simulink model "AC_grid_Dynamic"  (R2025a)
settings: Solver=VariableStepAuto  StartTime=0.0  StopTime=10.0  RelTol=1e-3
undefined symbols (not defined in the file): C_Lines, Cbuses, fref, From_buses, From_nodes, L_Loads, Lines_fromM, Lines_toM, Load_buses, Nbuses, R_Lines, R_Loads, shift_lines, tap_lines, To_buses, To_nodes
(part 1 of 2)
settings Model: Creator=atomas  LastModifiedBy=atomas

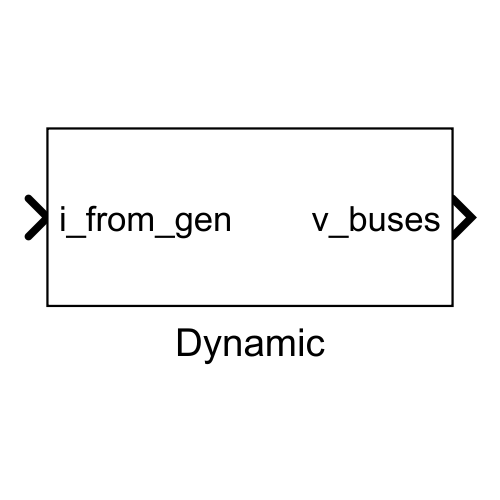
[thumbnail: Simulink's stored preview of the top-level diagram]
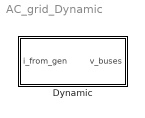
== system AC_grid_Dynamic ==
  Dynamic : Subsystem  VariantControl=Dynamic

== system AC_grid_Dynamic/Dynamic ==
  i_from_gen : Inport
  Buses : Subsystem
  Goto Tag Visibility : GotoTagVisibility  GotoTag=Cbuses
  Lines : Subsystem
  Lines to buses : Subsystem
  Loads : Subsystem
  Loads to buses : Subsystem
  Selector2 : Selector  NumberOfDimensions=2  InputPortWidth=Nnodes  IndexOptions=Select all,Index vector (dialog)  Indices=1,Load_buses  OutputSizes=1,1
  Selector4 : Selector  NumberOfDimensions=2  InputPortWidth=Nnodes  IndexOptions=Select all,Index vector (dialog)  Indices=From_nodes,From_buses  OutputSizes=1,1
  Selector6 : Selector  NumberOfDimensions=2  InputPortWidth=Nnodes  IndexOptions=Select all,Index vector (dialog)  Indices=To_nodes,To_buses  OutputSizes=1,1
  Step : Step  Before=ones(1, length(From_buses))  After=[1 ones(1, length(From_buses)-1)]  SampleTime=0
  Sum : Sum  Inputs=++|
  Sum1 : Sum  Inputs=|++
  connect : Subsystem
  iCbuses : Subsystem
  iP : Subsystem
  v_buses : Outport
  tag scope: Cbuses=scoped
  wires:
  iCbuses/1(Out1) -> [Cbuses]
  Lines/1(i) -> Lines to buses/1(i)
  Lines to buses/1(i_in_buses) -> [i_from_lines]
  Sum1/1 -> Buses/2(i_out)
  i_from_gen/1 -> Sum/1
  Step/1 -> Lines/3(connected), iCbuses/1(In1)
  [i_to_lines] -> Sum1/2
  [v_buses] -> Selector4/1
  Selector2/1 -> Loads/1(v_in)
  Selector4/1 -> Lines/1(v_in)
  Sum/1 -> Buses/1(i_in)
  Loads/1(i) -> Loads to buses/1(i_loads)
  [v_buses] -> Selector6/1
  connect/1(Out1) -> Loads/2(connected)
  [v_buses] -> Selector2/1
  Selector6/1 -> Lines/2(v_out)
  iP/1(Out1) -> Loads/3(iP)
  Loads to buses/1(i_out_buses) -> [i_to_loads]
  Lines to buses/2(i_out_buses) -> [i_to_lines]
  [i_to_loads] -> Sum1/1
  [i_from_lines] -> Sum/2
  Buses/1(v) -> v_buses/1, [v_buses]

== system AC_grid_Dynamic/Dynamic/Buses ==
  i_in : Inport
  i_out : Inport  Port=2
  Sum : Sum  Inputs=|++++
  dynamic : Subsystem  VariantControl=dynamic
  only R : Subsystem  Commented=on  VariantControl=only R
  static : Subsystem  Commented=on  VariantControl=static
  static omega : Subsystem  Commented=on  VariantControl=static omega
  v : Outport
  wires:
  Sum/1 -> v/1
  static/1(v) -> Sum/2
  only R/1(v) -> Sum/4
  i_in/1 -> dynamic/1(i_in), static/1(i_in), static omega/1(i_in), only R/1(i_in)
  dynamic/1(v) -> Sum/1
  i_out/1 -> dynamic/2(i_out), static/2(i_out), static omega/2(i_out), only R/2(i_out)
  static omega/1(v) -> Sum/3

== system AC_grid_Dynamic/Dynamic/Lines ==
  note: tap transformer
  v_in : Inport
  v_out : Inport  Port=2
  connected : Inport  Port=3
  Complex to Real-Imag : ComplexToRealImag
  Constant1 : Constant  Value=zeros(1, length(R_Lines))  VectorParams1D=off
  Gain : Gain  Gain=1./tap_lines.*(cos(shift_lines)-1i*sin(shift_lines))
  Matrix Concatenate : Concatenate  NumInputs=3  Mode=Multidimensional array
  Real-Imag to Complex : RealImagToComplex
  Selector : Selector  NumberOfDimensions=2  InputPortWidth=3  IndexOptions=Index vector (dialog),Select all  Indices=1,1  OutputSizes=1,1
  Selector1 : Selector  NumberOfDimensions=2  InputPortWidth=3  IndexOptions=Index vector (dialog),Select all  Indices=2,1  OutputSizes=1,1
  Sum : Sum  Inputs=|+++
  dynamic : Subsystem  VariantControl=dynamic
  static : Subsystem  Commented=on  VariantControl=static
  static omega : Subsystem  Commented=on  VariantControl=static_omega
  i : Outport
  wires:
  Real-Imag to Complex/1 -> Gain/1
  Gain/1 -> Complex to Real-Imag/1
  Selector1/1 -> Real-Imag to Complex/2
  Selector/1 -> Real-Imag to Complex/1
  Complex to Real-Imag/2 -> Matrix Concatenate/2
  Complex to Real-Imag/1 -> Matrix Concatenate/1
  Constant1/1 -> Matrix Concatenate/3
  v_in/1 -> Selector/1, Selector1/1
  Sum/1 -> i/1
  static omega/1(i) -> Sum/3
  static/1(i) -> Sum/2
  dynamic/1(i) -> Sum/1
  Matrix Concatenate/1 -> dynamic/1(v_in_d), static omega/1(v_in_d), static/1(v_in)
  v_out/1 -> dynamic/2(v_out), static/2(v_out_d), static omega/2(v_out)
  connected/1 -> dynamic/3(connected), static omega/3(connected), static/3(connected)

== system AC_grid_Dynamic/Dynamic/Lines to buses ==
  i : Inport
  Complex to Real-Imag : ComplexToRealImag
  Constant1 : Constant  Value=zeros(1, length(R_Lines))  VectorParams1D=off
  Gain : Gain  Gain=1./tap_lines.*(cos(shift_lines)-1i*sin(shift_lines))
  Lines_toM : Subsystem  TreatAsAtomicUnit=on
  Matrix Concatenate : Concatenate  NumInputs=3  Mode=Multidimensional array
  Real-Imag to Complex : RealImagToComplex
  Selector : Selector  NumberOfDimensions=2  InputPortWidth=3  IndexOptions=Index vector (dialog),Select all  Indices=1,1  OutputSizes=1,1
  Selector1 : Selector  NumberOfDimensions=2  InputPortWidth=3  IndexOptions=Index vector (dialog),Select all  Indices=2,1  OutputSizes=1,1
  i_in_buses : Outport
  i_out_buses : Outport  Port=2
  wires:
  Constant1/1 -> Matrix Concatenate/3
  Gain/1 -> Complex to Real-Imag/1
  Complex to Real-Imag/2 -> Matrix Concatenate/2
  Complex to Real-Imag/1 -> Matrix Concatenate/1
  Selector/1 -> Real-Imag to Complex/1
  Selector1/1 -> Real-Imag to Complex/2
  Real-Imag to Complex/1 -> Gain/1
  Matrix Concatenate/1 -> Lines_toM/2(i_from)
  Lines_toM/1(i_from_lines) -> i_in_buses/1
  i/1 -> Selector/1, Selector1/1, Lines_toM/1(i_to)
  Lines_toM/2(i_to_lines) -> i_out_buses/1

== system AC_grid_Dynamic/Dynamic/Loads ==
  v_in : Inport
  connected : Inport  Port=2
  iP : Inport  Port=3
  PQ : Subsystem  Commented=on  VariantControl=PQ
  Sum : Sum  Inputs=|++++++++
  dynamic PQ : Subsystem  Commented=on  VariantControl=dynamic_PQ
  parallel RL dynamic : Subsystem  Commented=on  VariantControl=dynamic
  parallel RL static : Subsystem  Commented=on  VariantControl=dynamic
  parallel RL static omega : Subsystem  Commented=on  VariantControl=dynamic
  series RL dynamic : Subsystem  Commented=on  VariantControl=dynamic
  series RL static : Subsystem  Commented=on  VariantControl=static
  series RL static omega : Subsystem  VariantControl=static_omega
  i : Outport
  wires:
  parallel RL static omega/1(i) -> Sum/8
  parallel RL static/1(i) -> Sum/7
  parallel RL dynamic/1(i) -> Sum/6
  Sum/1 -> i/1
  series RL static omega/1(i) -> Sum/3
  dynamic PQ/1(i) -> Sum/5
  PQ/1(i) -> Sum/4
  series RL static/1(i) -> Sum/2
  iP/1 -> dynamic PQ/3(iP), PQ/3(iP)
  connected/1 -> series RL static/1(connected), series RL static omega/2(connected), PQ/2(connected), dynamic PQ/2(connected), parallel RL static/2(connected), parallel RL static omega/2(connected), parallel RL dynamic/2(connected), series RL dynamic/2(connected)
  series RL dynamic/1(i) -> Sum/1
  v_in/1 -> series RL static/2(v_in), series RL static omega/1(v_in), PQ/1(v_in), dynamic PQ/1(v_in), parallel RL static/1(v_in), parallel RL static omega/1(v_in), parallel RL dynamic/1(v_in), series RL dynamic/1(v_in)

== system AC_grid_Dynamic/Dynamic/Loads to buses ==
  i_loads : Inport
  LoadsM : Subsystem  TreatAsAtomicUnit=on
  i_out_buses : Outport
  wires:
  LoadsM/1(Out1) -> i_out_buses/1
  i_loads/1 -> LoadsM/1(i)

== system AC_grid_Dynamic/Dynamic/connect ==
  note: in which load?
      | By default, the max(P)
  Assignment : Assignment  DiagnosticForDimensions=Warning  IndexOptions=Index vector (dialog)  Indices=1  OutputSizes=1
  One3 : Constant  Value=ones(1, length(L_Loads))  VectorParams1D=off  OutDataTypeStr=Inherit: Inherit via back propagation
  Step : Step  Before=1  SampleTime=0
  Out1 : Outport
  wires:
  Step/1 -> Assignment/2
  One3/1 -> Assignment/1
  Assignment/1 -> Out1/1

== system AC_grid_Dynamic/Dynamic/iCbuses ==
  In1 : Inport
  Constant : Constant  Value=Cbuses  VectorParams1D=off
  Constant1 : Constant  Value=C_Lines  VectorParams1D=off
  Gain : Gain  Gain=1/2
  Saturation : Saturate  UpperLimit=inf  LowerLimit=1e-3
  Subsystem : Subsystem
  Sum3 : Sum  Inputs=|-+
  Switch : Switch  Criteria=u2 > Threshold  SaturateOnIntegerOverflow=off  InputSameDT=off
  Zero : Constant  Value=zeros(1, length(From_buses))  VectorParams1D=off  OutDataTypeStr=Inherit: Inherit via back propagation
  Out1 : Outport
  wires:
  Subsystem/1(Out1) -> Sum3/1
  In1/1 -> Switch/2
  Constant1/1 -> Switch/3
  Gain/1 -> Subsystem/1(In1)
  Constant/1 -> Sum3/2
  Saturation/1 -> Out1/1
  Zero/1 -> Switch/1
  Sum3/1 -> Saturation/1
  Switch/1 -> Gain/1

== system AC_grid_Dynamic/Dynamic/iP ==
  note: in which load?
      | By default, the max(P)
  Assignment : Assignment  DiagnosticForDimensions=Warning  IndexOptions=Index vector (dialog)  Indices=find(Ploads == max(Ploads), 1)  OutputSizes=1
  Gain : Gain  Gain=0
  One3 : Constant  Value=zeros(1, length(L_Loads))  VectorParams1D=off  OutDataTypeStr=Inherit: Inherit via back propagation
  iP in % : Step  After=0.1  SampleTime=0  VectorParams1D=off  ZeroCross=off
  Out1 : Outport
  wires:
  Gain/1 -> Assignment/2
  Assignment/1 -> Out1/1
  iP in %/1 -> Gain/1
  One3/1 -> Assignment/1

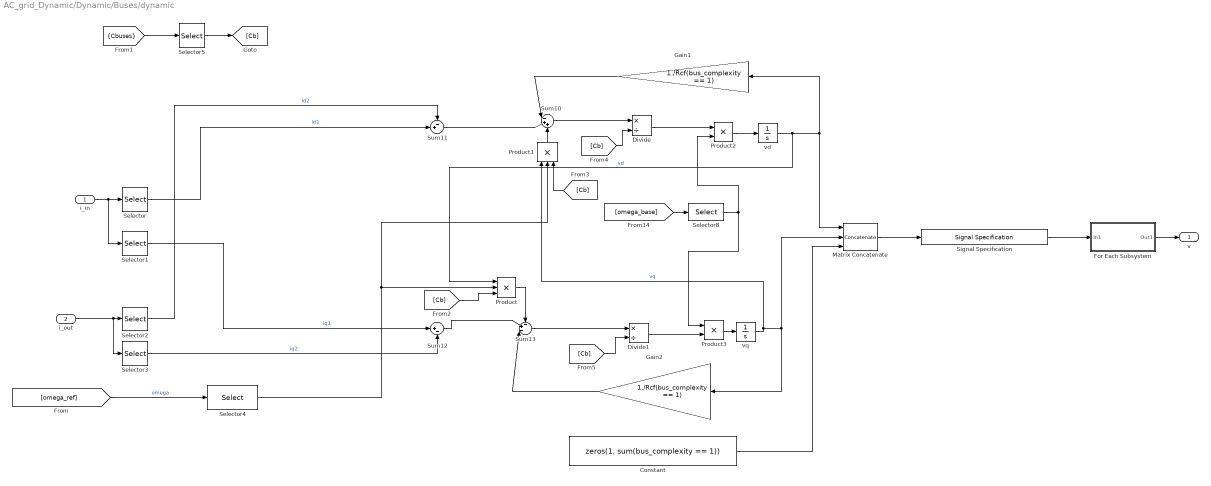
== system AC_grid_Dynamic/Dynamic/Buses/dynamic ==
  i_in : Inport
  i_out : Inport  Port=2
  Constant : Constant  Value=zeros(1, sum(bus_complexity == 1))  VectorParams1D=off
  Divide : Product  Inputs=*/
  Divide1 : Product  Inputs=*/
  For Each Subsystem : Subsystem  TreatAsAtomicUnit=on
  Gain1 : Gain  Gain=1./Rcf(bus_complexity == 1)
  Gain2 : Gain  Gain=1./Rcf(bus_complexity == 1)
  Matrix Concatenate : Concatenate  NumInputs=3  Mode=Multidimensional array
  Product : Product  Inputs=3
  Product1 : Product  Inputs=3
  Product2 : Product
  Product3 : Product
  Selector : Selector  NumberOfDimensions=2  InputPortWidth=3  IndexOptions=Index vector (dialog),Index vector (dialog)  Indices=1,find(bus_complexity == 1)  OutputSizes=1,1
  Selector1 : Selector  NumberOfDimensions=2  InputPortWidth=3  IndexOptions=Index vector (dialog),Index vector (dialog)  Indices=2,find(bus_complexity == 1)  OutputSizes=1,1
  Selector2 : Selector  NumberOfDimensions=2  InputPortWidth=3  IndexOptions=Index vector (dialog),Index vector (dialog)  Indices=1,find(bus_complexity == 1)  OutputSizes=1,1
  Selector3 : Selector  NumberOfDimensions=2  InputPortWidth=3  IndexOptions=Index vector (dialog),Index vector (dialog)  Indices=2,find(bus_complexity == 1)  OutputSizes=1,1
  Selector4 : Selector  InputPortWidth=length(fref.ref_units)  IndexOptions=Index vector (dialog)  Indices=fref.buses(bus_complexity == 1)  OutputSizes=1
  Selector5 : Selector  InputPortWidth=length(Cbuses)  IndexOptions=Index vector (dialog)  Indices=find(bus_complexity == 1)  OutputSizes=1
  Selector8 : Selector  InputPortWidth=length(fref.ref_units)  IndexOptions=Index vector (dialog)  Indices=fref.buses(bus_complexity == 1)  OutputSizes=1
  Signal Specification : SignalSpecification  Dimensions=[3 sum(bus_complexity == 1)]
  Sum10 : Sum  Inputs=|-++
  Sum11 : Sum  Inputs=-+|
  Sum12 : Sum  Inputs=|+-
  Sum13 : Sum  Inputs=-+-|
  vd : Integrator  InitialCondition=Grid_lf_op.op_report.Outputs(7).y(bus_complexity == 1)
  vq : Integrator  InitialCondition=Grid_lf_op.op_report.Outputs(8).y(bus_complexity == 1)
  v : Outport
  wires:
  Sum13/1 -> Divide1/1
  [Cb] -> Divide1/2
  [Cb] -> Divide/2
  [Cb] -> Product1/3
  [Cb] -> Product/3
  Selector5/1 -> [Cb]
  [Cbuses] -> Selector5/1
  Product3/1 -> vq/1
  Product2/1 -> vd/1
  Selector8/1 -> Product3/1, Product2/2
  [omega_base] -> Selector8/1
  Divide1/1 -> Product3/2
  Divide/1 -> Product2/1
  Selector4/1 -> Product/2, Product1/2
  Constant/1 -> Matrix Concatenate/3
  Signal Specification/1 -> For Each Subsystem/1(In1)
  For Each Subsystem/1(Out1) -> v/1
  Matrix Concatenate/1 -> Signal Specification/1
  i_out/1 -> Selector2/1, Selector3/1
  i_in/1 -> Selector1/1, Selector/1
  Selector3/1 -> Sum12/2  "iq2"
  Selector1/1 -> Sum12/1  "iq1"
  Selector2/1 -> Sum11/1  "id2"
  Selector/1 -> Sum11/2  "id1"
  vd/1 -> Product/1, Matrix Concatenate/1, Gain1/1  "vd"
  Sum12/1 -> Sum13/2
  Gain1/1 -> Sum10/1
  [omega_ref] -> Selector4/1  "omega"
  Sum11/1 -> Sum10/2
  Product/1 -> Sum13/1
  Gain2/1 -> Sum13/3
  Product1/1 -> Sum10/3
  vq/1 -> Matrix Concatenate/2, Gain2/1, Product1/1  "vq"
  Sum10/1 -> Divide/1

== system AC_grid_Dynamic/Dynamic/Buses/only R ==
  i_in : Inport
  i_out : Inport  Port=2
  Constant : Constant  Value=zeros(1, sum(bus_complexity == 4))  VectorParams1D=off
  For Each Subsystem : Subsystem  TreatAsAtomicUnit=on
  Gain : Gain  Gain=Rcf(bus_complexity == 4)
  Gain2 : Gain  Gain=Rcf(bus_complexity == 4)
  Matrix Concatenate : Concatenate  NumInputs=3  Mode=Multidimensional array
  Selector : Selector  NumberOfDimensions=2  InputPortWidth=3  IndexOptions=Index vector (dialog),Index vector (dialog)  Indices=1,find(bus_complexity == 4)  OutputSizes=1,1
  Selector1 : Selector  NumberOfDimensions=2  InputPortWidth=3  IndexOptions=Index vector (dialog),Index vector (dialog)  Indices=2,find(bus_complexity == 4)  OutputSizes=1,1
  Selector2 : Selector  NumberOfDimensions=2  InputPortWidth=3  IndexOptions=Index vector (dialog),Index vector (dialog)  Indices=1,find(bus_complexity == 4)  OutputSizes=1,1
  Selector3 : Selector  NumberOfDimensions=2  InputPortWidth=3  IndexOptions=Index vector (dialog),Index vector (dialog)  Indices=2,find(bus_complexity == 4)  OutputSizes=1,1
  Sum1 : Sum  Inputs=|+-
  Sum2 : Sum  Inputs=|+-
  v : Outport
  wires:
  Constant/1 -> Matrix Concatenate/3
  For Each Subsystem/1(Out1) -> v/1
  i_out/1 -> Selector3/1, Selector2/1
  Matrix Concatenate/1 -> For Each Subsystem/1(In1)
  i_in/1 -> Selector1/1, Selector/1
  Gain/1 -> Matrix Concatenate/1
  Gain2/1 -> Matrix Concatenate/2
  Selector2/1 -> Sum1/2
  Selector/1 -> Sum1/1  "id"
  Selector3/1 -> Sum2/2  "iq2"
  Sum2/1 -> Gain2/1  "iq"
  Sum1/1 -> Gain/1  "id"
  Selector1/1 -> Sum2/1  "iq1"

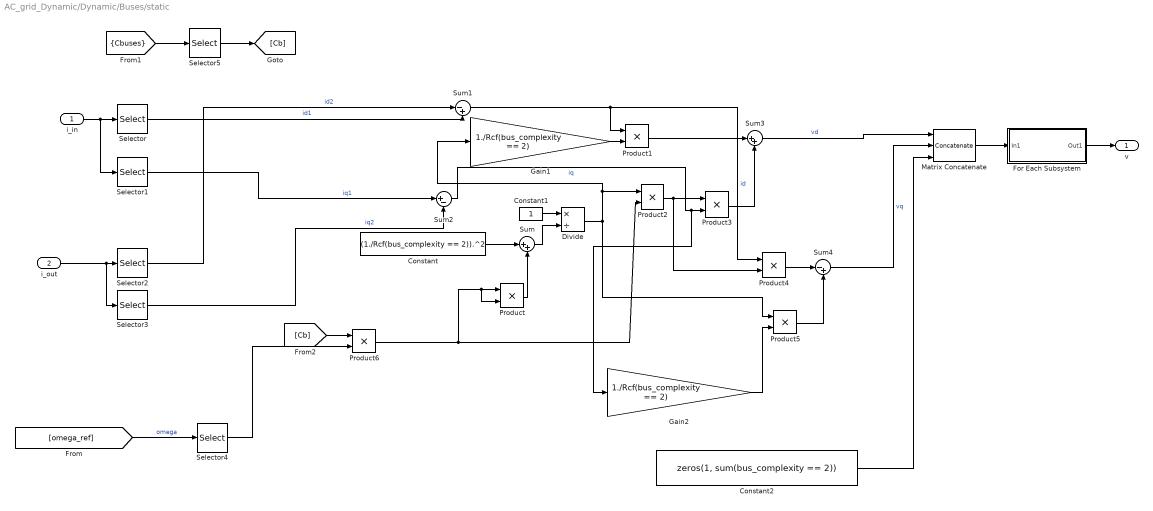
== system AC_grid_Dynamic/Dynamic/Buses/static ==
  i_in : Inport
  i_out : Inport  Port=2
  Constant : Constant  Value=(1./Rcf(bus_complexity == 2)).^2  VectorParams1D=off
  Constant1 : Constant
  Constant2 : Constant  Value=zeros(1, sum(bus_complexity == 2))  VectorParams1D=off
  Divide : Product  Inputs=*/
  For Each Subsystem : Subsystem  TreatAsAtomicUnit=on
  Gain1 : Gain  Gain=1./Rcf(bus_complexity == 2)
  Gain2 : Gain  Gain=1./Rcf(bus_complexity == 2)
  Matrix Concatenate : Concatenate  NumInputs=3  Mode=Multidimensional array
  Product{,1..6} (7 alike) : Product
  Selector : Selector  NumberOfDimensions=2  InputPortWidth=3  IndexOptions=Index vector (dialog),Index vector (dialog)  Indices=1,find(bus_complexity == 2)  OutputSizes=1,1
  Selector1 : Selector  NumberOfDimensions=2  InputPortWidth=3  IndexOptions=Index vector (dialog),Index vector (dialog)  Indices=2,find(bus_complexity == 2)  OutputSizes=1,1
  Selector2 : Selector  NumberOfDimensions=2  InputPortWidth=3  IndexOptions=Index vector (dialog),Index vector (dialog)  Indices=1,find(bus_complexity == 2)  OutputSizes=1,1
  Selector3 : Selector  NumberOfDimensions=2  InputPortWidth=3  IndexOptions=Index vector (dialog),Index vector (dialog)  Indices=2,find(bus_complexity == 2)  OutputSizes=1,1
  Selector4 : Selector  InputPortWidth=length(fref.ref_units)  IndexOptions=Index vector (dialog)  Indices=fref.buses(bus_complexity == 2)  OutputSizes=1
  Selector5 : Selector  InputPortWidth=length(Cbuses)  IndexOptions=Index vector (dialog)  Indices=find(bus_complexity == 2)  OutputSizes=1
  Sum : Sum  Inputs=|++
  Sum1 : Sum  Inputs=|-+
  Sum2 : Sum  Inputs=|+-
  Sum3 : Sum  Inputs=|++
  Sum4 : Sum  Inputs=|-+
  v : Outport
  wires:
  [Cb] -> Product6/1
  [Cbuses] -> Selector5/1
  Selector5/1 -> [Cb]
  Selector4/1 -> Product6/2
  Constant2/1 -> Matrix Concatenate/3
  For Each Subsystem/1(Out1) -> v/1
  i_out/1 -> Selector3/1, Selector2/1
  Matrix Concatenate/1 -> For Each Subsystem/1(In1)
  i_in/1 -> Selector1/1, Selector/1
  Selector3/1 -> Sum2/2  "iq2"
  Selector1/1 -> Sum2/1  "iq1"
  Selector2/1 -> Sum1/1  "id2"
  Selector/1 -> Sum1/2  "id1"
  [omega_ref] -> Selector4/1  "omega"
  Sum3/1 -> Matrix Concatenate/1  "vd"
  Sum4/1 -> Matrix Concatenate/2  "vq"
  Constant/1 -> Sum/1
  Sum/1 -> Divide/2
  Product6/1 -> Product2/2, Product/2, Product/1
  Product/1 -> Sum/2
  Constant1/1 -> Divide/1
  Sum1/1 -> Product1/1, Product4/1  "id"
  Sum2/1 -> Gain2/1, Product3/2  "iq"
  Gain1/1 -> Product1/2
  Divide/1 -> Product5/1, Gain1/1, Product2/1
  Product1/1 -> Sum3/1
  Product3/1 -> Sum3/2
  Product2/1 -> Product4/2, Product3/1
  Product4/1 -> Sum4/1
  Gain2/1 -> Product5/2
  Product5/1 -> Sum4/2

== system AC_grid_Dynamic/Dynamic/Buses/static omega ==
  i_in : Inport
  i_out : Inport  Port=2
  Constant : Constant  Value=zeros(1, sum(bus_complexity == 3))  VectorParams1D=off
  For Each Subsystem : Subsystem  TreatAsAtomicUnit=on
  Gain : Gain  Gain=1./((1./Rcf(bus_complexity == 3)).^2+Cbuses(bus_complexity == 3).^2)
  Gain1 : Gain  Gain=1./((1./Rcf(bus_complexity == 3)).^2+Cbuses(bus_complexity == 3).^2)
  Gain3 : Gain  Gain=1./Rcf(bus_complexity == 3)
  Gain5 : Gain  Gain=1./Rcf(bus_complexity == 3)
  IC : InitialCondition  Value=[Grid_lf_op.op_report.Outputs(7).y(bus_complexity == 3); Grid_lf_op.op_report.Outputs(8).y(bus_complexity == 3); 0*Grid_lf_op.op_report.Outputs(7).y(bus_complexity == 3)]
  LPF : Subsystem  Commented=through
  Matrix Concatenate : Concatenate  NumInputs=3  Mode=Multidimensional array
  Product : Product
  Product1 : Product
  Selector : Selector  NumberOfDimensions=2  InputPortWidth=3  IndexOptions=Index vector (dialog),Index vector (dialog)  Indices=1,find(bus_complexity == 3)  OutputSizes=1,1
  Selector1 : Selector  NumberOfDimensions=2  InputPortWidth=3  IndexOptions=Index vector (dialog),Index vector (dialog)  Indices=2,find(bus_complexity == 3)  OutputSizes=1,1
  Selector2 : Selector  NumberOfDimensions=2  InputPortWidth=3  IndexOptions=Index vector (dialog),Index vector (dialog)  Indices=1,find(bus_complexity == 3)  OutputSizes=1,1
  Selector3 : Selector  NumberOfDimensions=2  InputPortWidth=3  IndexOptions=Index vector (dialog),Index vector (dialog)  Indices=2,find(bus_complexity == 3)  OutputSizes=1,1
  Selector5 : Selector  InputPortWidth=length(Cbuses)  IndexOptions=Index vector (dialog)  Indices=find(bus_complexity == 3)  OutputSizes=1
  Sum : Sum  Inputs=|++
  Sum1 : Sum  Inputs=|+-
  Sum2 : Sum  Inputs=|+-
  Sum4 : Sum  Inputs=|-+
  v : Outport
  wires:
  [Cb] -> Product1/2
  [Cb] -> Product/2
  [Cbuses] -> Selector5/1
  Selector5/1 -> [Cb]
  IC/1 -> For Each Subsystem/1(In1)
  LPF/1(out) -> IC/1
  Matrix Concatenate/1 -> LPF/1(in)
  Constant/1 -> Matrix Concatenate/3
  For Each Subsystem/1(Out1) -> v/1
  i_out/1 -> Selector2/1, Selector3/1
  i_in/1 -> Selector/1, Selector1/1
  Sum/1 -> Matrix Concatenate/1
  Sum4/1 -> Matrix Concatenate/2
  Gain5/1 -> Sum4/2
  Product/1 -> Sum4/1
  Product1/1 -> Sum/2
  Gain3/1 -> Sum/1
  Gain1/1 -> Gain5/1, Product1/1
  Gain/1 -> Gain3/1, Product/1
  Selector2/1 -> Sum1/2
  Selector/1 -> Sum1/1  "id"
  Selector3/1 -> Sum2/2  "iq2"
  Sum2/1 -> Gain1/1  "iq"
  Sum1/1 -> Gain/1  "id"
  Selector1/1 -> Sum2/1  "iq1"

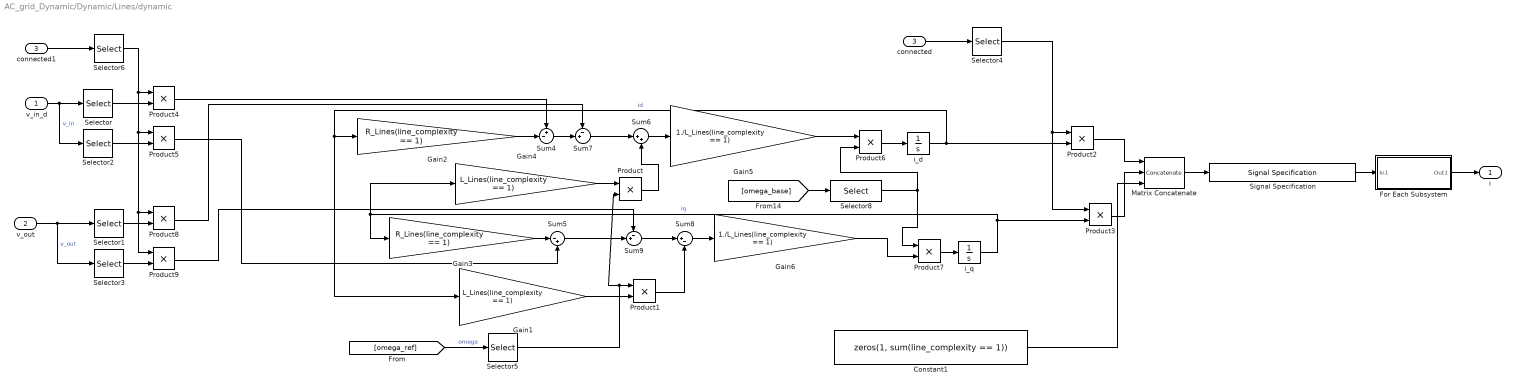
== system AC_grid_Dynamic/Dynamic/Lines/dynamic ==
  v_in_d : Inport
  v_out : Inport  Port=2
  connected : Inport  Port=3
  Constant1 : Constant  Value=zeros(1, sum(line_complexity == 1))  VectorParams1D=off
  For Each Subsystem : Subsystem  TreatAsAtomicUnit=on
  Gain1 : Gain  Gain=L_Lines(line_complexity == 1)
  Gain2 : Gain  Gain=R_Lines(line_complexity == 1)
  Gain3 : Gain  Gain=R_Lines(line_complexity == 1)
  Gain4 : Gain  Gain=L_Lines(line_complexity == 1)
  Gain5 : Gain  Gain=1./L_Lines(line_complexity == 1)
  Gain6 : Gain  Gain=1./L_Lines(line_complexity == 1)
  Matrix Concatenate : Concatenate  NumInputs=3  Mode=Multidimensional array
  Product{,1..9} (10 alike) : Product
  Selector : Selector  NumberOfDimensions=2  InputPortWidth=3  IndexOptions=Index vector (dialog),Index vector (dialog)  Indices=1,find(line_complexity == 1)  OutputSizes=1,1
  Selector1 : Selector  NumberOfDimensions=2  InputPortWidth=3  IndexOptions=Index vector (dialog),Index vector (dialog)  Indices=1,find(line_complexity == 1)  OutputSizes=1,1
  Selector2 : Selector  NumberOfDimensions=2  InputPortWidth=3  IndexOptions=Index vector (dialog),Index vector (dialog)  Indices=2,find(line_complexity == 1)  OutputSizes=1,1
  Selector3 : Selector  NumberOfDimensions=2  InputPortWidth=3  IndexOptions=Index vector (dialog),Index vector (dialog)  Indices=2,find(line_complexity == 1)  OutputSizes=1,1
  Selector4 : Selector  InputPortWidth=length(From_buses)  IndexOptions=Index vector (dialog)  Indices=find(line_complexity == 1)  OutputSizes=1
  Selector5 : Selector  InputPortWidth=length(fref.ref_units)  IndexOptions=Index vector (dialog)  Indices=fref.lines(line_complexity == 1)  OutputSizes=1
  Selector6 : Selector  InputPortWidth=length(From_buses)  IndexOptions=Index vector (dialog)  Indices=find(line_complexity == 1)  OutputSizes=1
  Selector8 : Selector  InputPortWidth=length(fref.ref_units)  IndexOptions=Index vector (dialog)  Indices=fref.lines(line_complexity == 1)  OutputSizes=1
  Signal Specification : SignalSpecification  Dimensions=[3 sum(line_complexity == 1)]
  Sum4 : Sum  Inputs=+-|
  Sum5 : Sum  Inputs=|-+
  Sum6 : Sum  Inputs=|++
  Sum7 : Sum  Inputs=-+|
  Sum8 : Sum  Inputs=|+-
  Sum9 : Sum  Inputs=-+|
  connected1 : InportShadow  Port=3
  i_d : Integrator  InitialCondition=Grid_lf_op.op_report.Outputs(3).y(line_complexity == 1)
  i_q : Integrator  InitialCondition=Grid_lf_op.op_report.Outputs(4).y(line_complexity == 1)
  i : Outport
  wires:
  Selector3/1 -> Product9/2
  Selector1/1 -> Product8/2
  Selector2/1 -> Product5/2
  Selector6/1 -> Product4/1, Product5/1, Product8/1, Product9/1
  Selector/1 -> Product4/2
  connected1/1 -> Selector6/1
  Product7/1 -> i_q/1
  Product6/1 -> i_d/1
  Gain6/1 -> Product7/2
  Gain5/1 -> Product6/1
  [omega_base] -> Selector8/1
  Selector8/1 -> Product7/1, Product6/2
  Selector5/1 -> Product1/1, Product/2
  Constant1/1 -> Matrix Concatenate/3
  Signal Specification/1 -> For Each Subsystem/1(In1)
  For Each Subsystem/1(Out1) -> i/1
  Selector4/1 -> Product2/1, Product3/1
  Product9/1 -> Sum9/1
  Product8/1 -> Sum7/1
  Product4/1 -> Sum4/1
  Product3/1 -> Matrix Concatenate/2
  Product2/1 -> Matrix Concatenate/1
  Matrix Concatenate/1 -> Signal Specification/1
  connected/1 -> Selector4/1
  Product5/1 -> Sum5/2
  v_in_d/1 -> Selector/1, Selector2/1  "v_in"
  Gain2/1 -> Sum4/2
  i_d/1 -> Product2/2, Gain2/1, Gain1/1  "id"
  Sum6/1 -> Gain5/1
  [omega_ref] -> Selector5/1  "omega"
  Product/1 -> Sum6/2
  Sum8/1 -> Gain6/1
  Sum4/1 -> Sum7/2
  Product1/1 -> Sum8/2
  Gain4/1 -> Product/1
  Sum7/1 -> Sum6/1
  Gain3/1 -> Sum5/1
  Sum5/1 -> Sum9/2
  i_q/1 -> Product3/2, Gain4/1, Gain3/1  "iq"
  Gain1/1 -> Product1/2
  Sum9/1 -> Sum8/1
  v_out/1 -> Selector1/1, Selector3/1  "v_out"

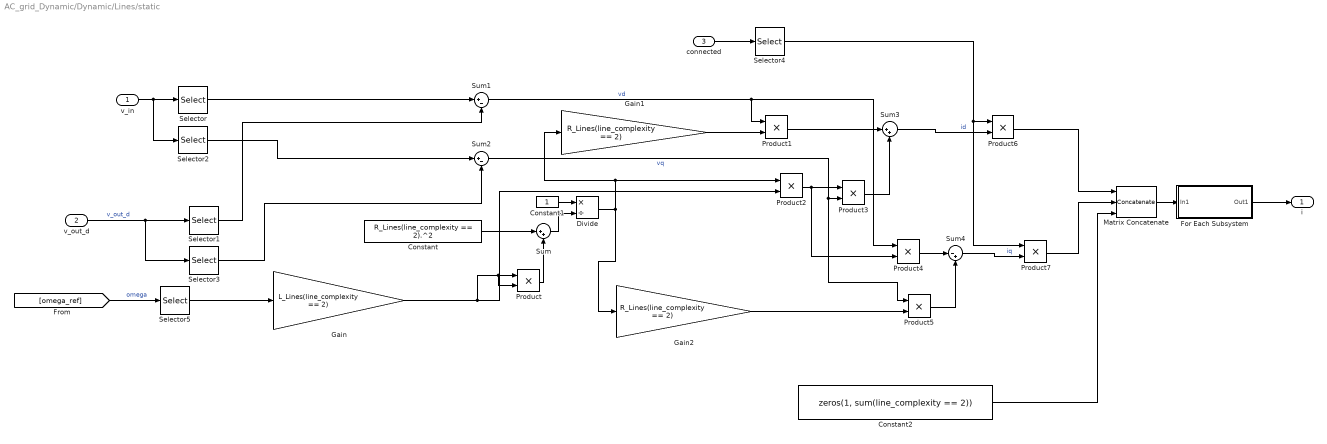
== system AC_grid_Dynamic/Dynamic/Lines/static ==
  v_in : Inport
  v_out_d : Inport  Port=2
  connected : Inport  Port=3
  Constant : Constant  Value=R_Lines(line_complexity == 2).^2  VectorParams1D=off
  Constant1 : Constant
  Constant2 : Constant  Value=zeros(1, sum(line_complexity == 2))  VectorParams1D=off
  Divide : Product  Inputs=*/
  For Each Subsystem : Subsystem  TreatAsAtomicUnit=on
  Gain : Gain  Gain=L_Lines(line_complexity == 2)
  Gain1 : Gain  Gain=R_Lines(line_complexity == 2)
  Gain2 : Gain  Gain=R_Lines(line_complexity == 2)
  Matrix Concatenate : Concatenate  NumInputs=3  Mode=Multidimensional array
  Product{,1..7} (8 alike) : Product
  Selector : Selector  NumberOfDimensions=2  InputPortWidth=3  IndexOptions=Index vector (dialog),Index vector (dialog)  Indices=1,find(line_complexity == 2)  OutputSizes=1,1
  Selector1 : Selector  NumberOfDimensions=2  InputPortWidth=3  IndexOptions=Index vector (dialog),Index vector (dialog)  Indices=1,find(line_complexity == 2)  OutputSizes=1,1
  Selector2 : Selector  NumberOfDimensions=2  InputPortWidth=3  IndexOptions=Index vector (dialog),Index vector (dialog)  Indices=2,find(line_complexity == 2)  OutputSizes=1,1
  Selector3 : Selector  NumberOfDimensions=2  InputPortWidth=3  IndexOptions=Index vector (dialog),Index vector (dialog)  Indices=2,find(line_complexity == 2)  OutputSizes=1,1
  Selector4 : Selector  InputPortWidth=length(From_buses)  IndexOptions=Index vector (dialog)  Indices=find(line_complexity == 2)  OutputSizes=1
  Selector5 : Selector  InputPortWidth=length(fref.ref_units)  IndexOptions=Index vector (dialog)  Indices=fref.lines(line_complexity == 2)  OutputSizes=1
  Sum : Sum  Inputs=|++
  Sum1 : Sum  Inputs=|+-
  Sum2 : Sum  Inputs=|+-
  Sum3 : Sum  Inputs=|++
  Sum4 : Sum  Inputs=|-+
  i : Outport
  wires:
  Selector5/1 -> Gain/1
  Constant2/1 -> Matrix Concatenate/3
  For Each Subsystem/1(Out1) -> i/1
  Selector4/1 -> Product6/1, Product7/1
  Product7/1 -> Matrix Concatenate/2
  Product6/1 -> Matrix Concatenate/1
  Matrix Concatenate/1 -> For Each Subsystem/1(In1)
  Selector/1 -> Sum1/1
  Selector2/1 -> Sum2/1
  Selector3/1 -> Sum2/2
  Selector1/1 -> Sum1/2
  connected/1 -> Selector4/1
  v_in/1 -> Selector/1, Selector2/1
  v_out_d/1 -> Selector1/1, Selector3/1  "v_out_d"
  Sum/1 -> Divide/2
  Gain2/1 -> Product5/2
  Product/1 -> Sum/2
  Product1/1 -> Sum3/1
  Product5/1 -> Sum4/2
  Constant/1 -> Sum/1
  Sum2/1 -> Product3/2, Product5/1  "vq"
  Gain/1 -> Product/1, Product/2, Product2/2
  Constant1/1 -> Divide/1
  Product3/1 -> Sum3/2
  Sum1/1 -> Product4/1, Product1/1  "vd"
  Divide/1 -> Product2/1, Gain1/1, Gain2/1
  Product4/1 -> Sum4/1
  Product2/1 -> Product3/1, Product4/2
  Gain1/1 -> Product1/2
  Sum3/1 -> Product6/2  "id"
  Sum4/1 -> Product7/2  "iq"
  [omega_ref] -> Selector5/1  "omega"

== system AC_grid_Dynamic/Dynamic/Lines/static omega ==
  v_in_d : Inport
  v_out : Inport  Port=2
  connected : Inport  Port=3
  Constant1 : Constant  Value=zeros(1, sum(line_complexity == 3))  VectorParams1D=off
  For Each Subsystem : Subsystem  TreatAsAtomicUnit=on
  Gain : Gain  Gain=1./(R_Lines(line_complexity == 3).^2+L_Lines(line_complexity == 3).^2)
  Gain1 : Gain  Gain=1./(R_Lines(line_complexity == 3).^2+L_Lines(line_complexity == 3).^2)
  Gain3 : Gain  Gain=R_Lines(line_complexity == 3)
  Gain4 : Gain  Gain=L_Lines(line_complexity == 3)
  Gain5 : Gain  Gain=L_Lines(line_complexity == 3)
  Gain6 : Gain  Gain=R_Lines(line_complexity == 3)
  Matrix Concatenate : Concatenate  NumInputs=3  Mode=Multidimensional array
  Product2 : Product
  Product3 : Product
  Selector : Selector  NumberOfDimensions=2  InputPortWidth=3  IndexOptions=Index vector (dialog),Index vector (dialog)  Indices=1,find(line_complexity == 3)  OutputSizes=1,1
  Selector1 : Selector  NumberOfDimensions=2  InputPortWidth=3  IndexOptions=Index vector (dialog),Index vector (dialog)  Indices=1,find(line_complexity == 3)  OutputSizes=1,1
  Selector2 : Selector  NumberOfDimensions=2  InputPortWidth=3  IndexOptions=Index vector (dialog),Index vector (dialog)  Indices=2,find(line_complexity == 3)  OutputSizes=1,1
  Selector3 : Selector  NumberOfDimensions=2  InputPortWidth=3  IndexOptions=Index vector (dialog),Index vector (dialog)  Indices=2,find(line_complexity == 3)  OutputSizes=1,1
  Selector4 : Selector  InputPortWidth=length(From_buses)  IndexOptions=Index vector (dialog)  Indices=find(line_complexity == 3)  OutputSizes=1
  Sum : Sum  Inputs=|++
  Sum1 : Sum  Inputs=|+-
  Sum2 : Sum  Inputs=|+-
  Sum3 : Sum  Inputs=|-+
  i : Outport
  wires:
  Constant1/1 -> Matrix Concatenate/3
  For Each Subsystem/1(Out1) -> i/1
  Selector4/1 -> Product2/1, Product3/1
  Selector1/1 -> Sum1/2
  v_out/1 -> Selector1/1, Selector3/1
  Selector2/1 -> Sum2/1
  Selector/1 -> Sum1/1
  v_in_d/1 -> Selector/1, Selector2/1  "v_in"
  Product3/1 -> Matrix Concatenate/2
  Product2/1 -> Matrix Concatenate/1
  Matrix Concatenate/1 -> For Each Subsystem/1(In1)
  connected/1 -> Selector4/1
  Gain6/1 -> Sum3/2
  Sum3/1 -> Product3/2
  Gain5/1 -> Sum3/1
  Sum/1 -> Product2/2
  Gain1/1 -> Gain6/1, Gain4/1
  Gain4/1 -> Sum/2
  Gain3/1 -> Sum/1
  Gain/1 -> Gain5/1, Gain3/1
  Sum2/1 -> Gain1/1  "vq"
  Sum1/1 -> Gain/1  "vd"
  Selector3/1 -> Sum2/2  "v_out_q"

== system AC_grid_Dynamic/Dynamic/Lines to buses/Lines_toM ==
  i_to : Inport  Partition=on  PartitionDimension=1  PartitionWidth=1  PartitionOffset=0
  i_from : Inport  Port=2  Partition=on  PartitionDimension=1  PartitionWidth=1  PartitionOffset=0
  For Each : ForEach  DisableCoverage=on
  State-Space : StateSpace  A=[]  B=[]  C=[]  D=Lines_toM  InitialCondition=0  ParameterTunability=Optimized
  State-Space1 : StateSpace  A=[]  B=[]  C=[]  D=Lines_fromM  InitialCondition=0  ParameterTunability=Optimized
  Transpose{,1..3} (4 alike) : Math  Operator=transpose
  i_from_lines : Outport  ConcatenationDimension=1
  i_to_lines : Outport  Port=2  ConcatenationDimension=1
  wires:
  Transpose3/1 -> i_to_lines/1
  i_from/1 -> Transpose2/1
  State-Space1/1 -> Transpose3/1
  Transpose2/1 -> State-Space1/1
  Transpose/1 -> State-Space/1
  State-Space/1 -> Transpose1/1
  i_to/1 -> Transpose/1
  Transpose1/1 -> i_from_lines/1

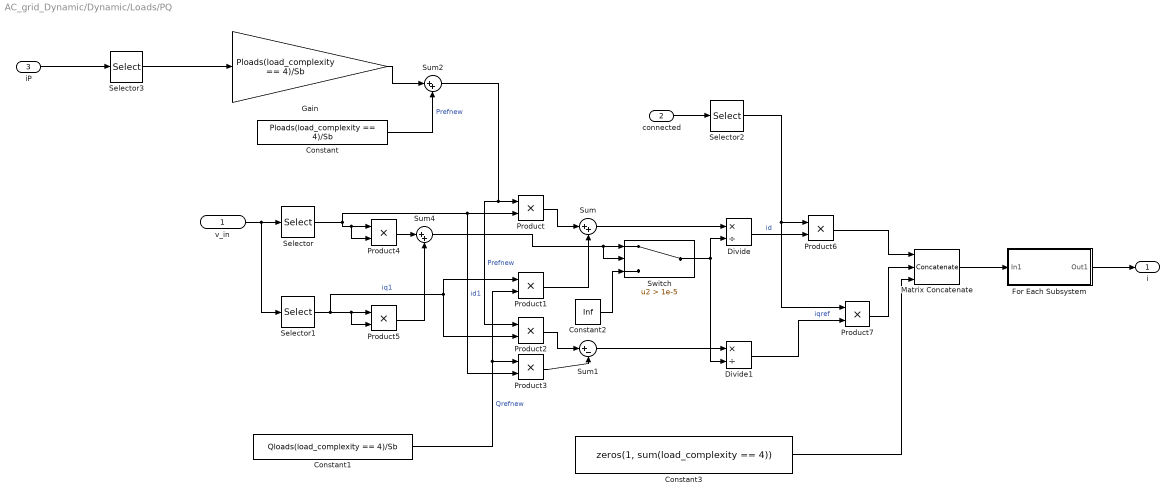
== system AC_grid_Dynamic/Dynamic/Loads/PQ ==
  v_in : Inport
  connected : Inport  Port=2
  iP : Inport  Port=3
  Constant : Constant  Value=Ploads(load_complexity == 4)/Sb  VectorParams1D=off
  Constant1 : Constant  Value=Qloads(load_complexity == 4)/Sb  VectorParams1D=off
  Constant2 : Constant  Value=Inf
  Constant3 : Constant  Value=zeros(1, sum(load_complexity == 4))  VectorParams1D=off
  Divide : Product  Inputs=*/
  Divide1 : Product  Inputs=*/
  For Each Subsystem : Subsystem  TreatAsAtomicUnit=on
  Gain : Gain  Gain=Ploads(load_complexity == 4)/Sb
  Matrix Concatenate : Concatenate  NumInputs=3  Mode=Multidimensional array
  Product{,1..7} (8 alike) : Product
  Selector : Selector  NumberOfDimensions=2  InputPortWidth=3  IndexOptions=Index vector (dialog),Index vector (dialog)  Indices=1,find(load_complexity == 4)  OutputSizes=1,1
  Selector1 : Selector  NumberOfDimensions=2  InputPortWidth=3  IndexOptions=Index vector (dialog),Index vector (dialog)  Indices=2,find(load_complexity == 4)  OutputSizes=1,1
  Selector2 : Selector  InputPortWidth=length(R_Loads)  IndexOptions=Index vector (dialog)  Indices=find(load_complexity == 4)  OutputSizes=1
  Selector3 : Selector  InputPortWidth=length(R_Loads)  IndexOptions=Index vector (dialog)  Indices=find(load_complexity == 4)  OutputSizes=1
  Sum : Sum  Inputs=|++
  Sum1 : Sum  Inputs=|+-
  Sum2 : Sum  Inputs=|++
  Sum4 : Sum  Inputs=|++
  Switch : Switch  Criteria=u2 > Threshold  Threshold=1e-5  ZeroCross=off  SaturateOnIntegerOverflow=off  InputSameDT=off
  i : Outport
  wires:
  Constant/1 -> Sum2/2  "Prefnew"
  iP/1 -> Selector3/1
  Gain/1 -> Sum2/1
  Selector3/1 -> Gain/1
  Constant3/1 -> Matrix Concatenate/3
  For Each Subsystem/1(Out1) -> i/1
  Selector2/1 -> Product7/1, Product6/1
  Product7/1 -> Matrix Concatenate/2
  Product6/1 -> Matrix Concatenate/1
  Matrix Concatenate/1 -> For Each Subsystem/1(In1)
  Selector1/1 -> Product1/1, Product2/2, Product5/2, Product5/1  "iq1"
  Selector/1 -> Product3/2, Product/2, Product4/2, Product4/1  "id1"
  Divide1/1 -> Product7/2  "iqref"
  Divide/1 -> Product6/2  "id"
  connected/1 -> Selector2/1
  Sum1/1 -> Divide1/1
  Constant2/1 -> Switch/3
  Sum4/1 -> Switch/2, Switch/1
  Switch/1 -> Divide/2, Divide1/2
  Sum/1 -> Divide/1
  Product4/1 -> Sum4/1
  Constant1/1 -> Product1/2, Product3/1  "Qrefnew"
  Product5/1 -> Sum4/2
  Product3/1 -> Sum1/2
  v_in/1 -> Selector/1, Selector1/1
  Product2/1 -> Sum1/1
  Sum2/1 -> Product2/1, Product/1  "Prefnew"
  Product/1 -> Sum/1
  Product1/1 -> Sum/2

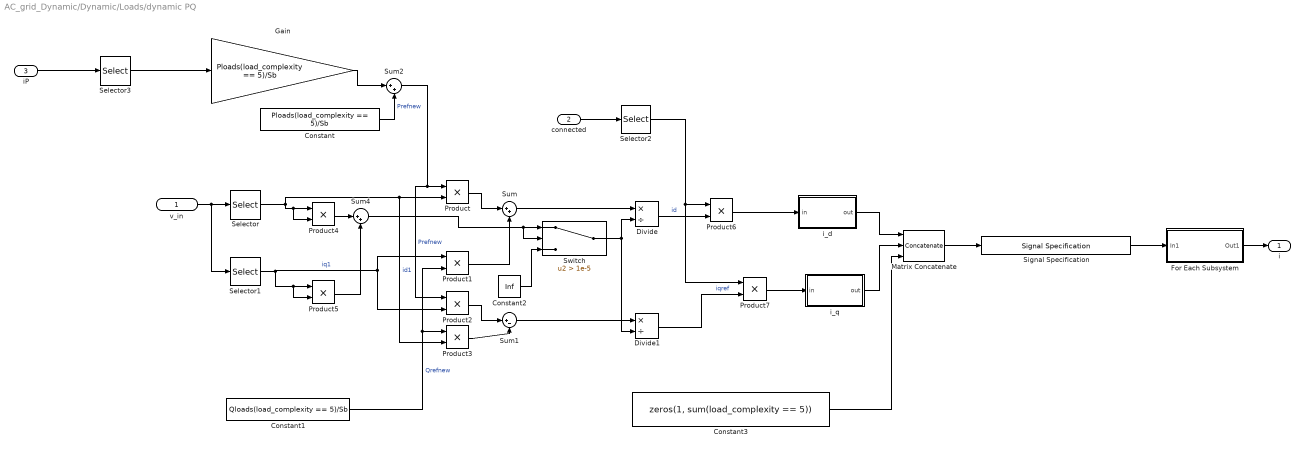
== system AC_grid_Dynamic/Dynamic/Loads/dynamic PQ ==
  v_in : Inport
  connected : Inport  Port=2
  iP : Inport  Port=3
  Constant : Constant  Value=Ploads(load_complexity == 5)/Sb  VectorParams1D=off
  Constant1 : Constant  Value=Qloads(load_complexity == 5)/Sb  VectorParams1D=off
  Constant2 : Constant  Value=Inf
  Constant3 : Constant  Value=zeros(1, sum(load_complexity == 5))  VectorParams1D=off
  Divide : Product  Inputs=*/
  Divide1 : Product  Inputs=*/
  For Each Subsystem : Subsystem  TreatAsAtomicUnit=on
  Gain : Gain  Gain=Ploads(load_complexity == 5)/Sb
  Matrix Concatenate : Concatenate  NumInputs=3  Mode=Multidimensional array
  Product{,1..7} (8 alike) : Product
  Selector : Selector  NumberOfDimensions=2  InputPortWidth=3  IndexOptions=Index vector (dialog),Index vector (dialog)  Indices=1,find(load_complexity == 5)  OutputSizes=1,1
  Selector1 : Selector  NumberOfDimensions=2  InputPortWidth=3  IndexOptions=Index vector (dialog),Index vector (dialog)  Indices=2,find(load_complexity == 5)  OutputSizes=1,1
  Selector2 : Selector  InputPortWidth=length(R_Loads)  IndexOptions=Index vector (dialog)  Indices=find(load_complexity == 5)  OutputSizes=1
  Selector3 : Selector  InputPortWidth=length(R_Loads)  IndexOptions=Index vector (dialog)  Indices=find(load_complexity == 5)  OutputSizes=1
  Signal Specification : SignalSpecification  Dimensions=[3 sum(load_complexity == 5)]
  Sum : Sum  Inputs=|++
  Sum1 : Sum  Inputs=|+-
  Sum2 : Sum  Inputs=|++
  Sum4 : Sum  Inputs=|++
  Switch : Switch  Criteria=u2 > Threshold  Threshold=1e-5  ZeroCross=off  SaturateOnIntegerOverflow=off  InputSameDT=off
  i_d : Subsystem  mask{T_s=0.01}
      mask prompts: T_s "Filter time constant"
      mask Display:
      | try
      |     dpoly(1, [T_s, 1])
      | catch
      | end
  i_q : Subsystem  mask{T_s=0.01}
      mask prompts: T_s "Filter time constant"
      mask Display:
      | try
      |     dpoly(1, [T_s, 1])
      | catch
      | end
  i : Outport
  wires:
  Constant3/1 -> Matrix Concatenate/3
  Signal Specification/1 -> For Each Subsystem/1(In1)
  For Each Subsystem/1(Out1) -> i/1
  Selector3/1 -> Gain/1
  Selector2/1 -> Product6/1, Product7/1
  i_q/1(out) -> Matrix Concatenate/2
  i_d/1(out) -> Matrix Concatenate/1
  Matrix Concatenate/1 -> Signal Specification/1
  Selector1/1 -> Product5/1, Product5/2, Product2/2, Product1/1  "iq1"
  Selector/1 -> Product4/1, Product4/2, Product/2, Product3/2  "id1"
  Constant1/1 -> Product3/1, Product1/2  "Qrefnew"
  Gain/1 -> Sum2/1
  Constant/1 -> Sum2/2  "Prefnew"
  iP/1 -> Selector3/1
  Product1/1 -> Sum/2
  Product/1 -> Sum/1
  Sum2/1 -> Product/1, Product2/1  "Prefnew"
  Product2/1 -> Sum1/1
  v_in/1 -> Selector1/1, Selector/1
  Product3/1 -> Sum1/2
  Product5/1 -> Sum4/2
  Product4/1 -> Sum4/1
  Sum/1 -> Divide/1
  Switch/1 -> Divide1/2, Divide/2
  Sum4/1 -> Switch/1, Switch/2
  Constant2/1 -> Switch/3
  Sum1/1 -> Divide1/1
  connected/1 -> Selector2/1
  Divide/1 -> Product6/2  "id"
  Product6/1 -> i_d/1(in)
  Divide1/1 -> Product7/2  "iqref"
  Product7/1 -> i_q/1(in)

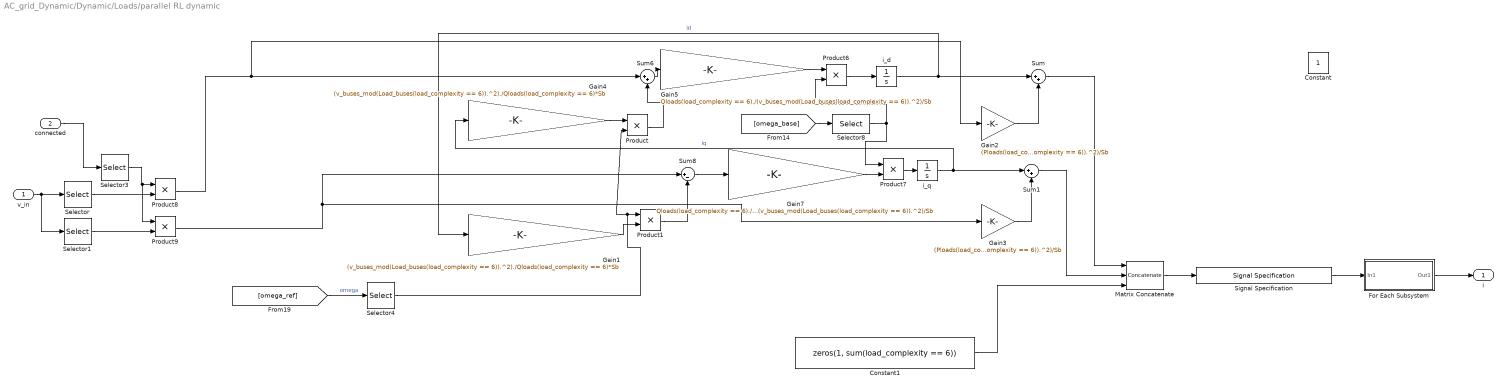
== system AC_grid_Dynamic/Dynamic/Loads/parallel RL dynamic ==
  v_in : Inport
  connected : Inport  Port=2
  Constant : Constant
  Constant1 : Constant  Value=zeros(1, sum(load_complexity == 6))  VectorParams1D=off
  For Each Subsystem : Subsystem  TreatAsAtomicUnit=on
  Gain1 : Gain  Gain=(v_buses_mod(Load_buses(load_complexity == 6)).^2)./Qloads(load_complexity == 6)*Sb
  Gain2 : Gain  Gain=(Ploads(load_complexity == 6)./v_buses_mod(Load_buses(load_complexity == 6)).^2)/Sb
  Gain3 : Gain  Gain=(Ploads(load_complexity == 6)./v_buses_mod(Load_buses(load_complexity == 6)).^2)/Sb
  Gain4 : Gain  Gain=(v_buses_mod(Load_buses(load_complexity == 6)).^2)./Qloads(load_complexity == 6)*Sb
  Gain5 : Gain  Gain=Qloads(load_complexity == 6)./(v_buses_mod(Load_buses(load_complexity == 6)).^2)/Sb
  Gain7 : Gain  Gain=Qloads(load_complexity == 6)./(v_buses_mod(Load_buses(load_complexity == 6)).^2)/Sb
  Matrix Concatenate : Concatenate  NumInputs=3  Mode=Multidimensional array
  Product{,1,6..9} (6 alike) : Product
  Selector : Selector  NumberOfDimensions=2  InputPortWidth=3  IndexOptions=Index vector (dialog),Index vector (dialog)  Indices=1,find(load_complexity == 6)  OutputSizes=1,1
  Selector1 : Selector  NumberOfDimensions=2  InputPortWidth=3  IndexOptions=Index vector (dialog),Index vector (dialog)  Indices=2,find(load_complexity == 6)  OutputSizes=1,1
  Selector3 : Selector  InputPortWidth=length(R_Loads)  IndexOptions=Index vector (dialog)  Indices=find(load_complexity == 6)  OutputSizes=1
  Selector4 : Selector  InputPortWidth=length(fref.ref_units)  IndexOptions=Index vector (dialog)  Indices=fref.loads(load_complexity == 6)  OutputSizes=1
  Selector8 : Selector  InputPortWidth=length(fref.ref_units)  IndexOptions=Index vector (dialog)  Indices=fref.loads(load_complexity == 6)  OutputSizes=1
  Signal Specification : SignalSpecification  Dimensions=[3 sum(load_complexity == 6)]
  Sum : Sum  Inputs=|++
  Sum1 : Sum  Inputs=|++
  Sum6 : Sum  Inputs=|++
  Sum8 : Sum  Inputs=|+-
  i_d : Integrator  InitialCondition=Grid_lf_op.op_report.Outputs(8).y(Load_buses(load_complexity == 6)).*Qloads(load_complexity == 6)./(v_buses_mod(Load_buses(load_complexity == 6)).^2)/Sb
  i_q : Integrator  InitialCondition=Grid_lf_op.op_report.Outputs(7).y(Load_buses(load_complexity == 6)).*-Qloads(load_complexity == 6)./(v_buses_mod(Load_buses(load_complexity == 6)).^2)/Sb
  i : Outport
  wires:
  Sum1/1 -> Matrix Concatenate/2
  Gain3/1 -> Sum1/2
  Gain2/1 -> Sum/2
  Sum/1 -> Matrix Concatenate/1
  Gain5/1 -> Product6/1
  Matrix Concatenate/1 -> Signal Specification/1
  Product8/1 -> Sum6/1, Gain2/1
  Product9/1 -> Sum8/1, Gain3/1
  Selector8/1 -> Product6/2, Product7/1
  Product/1 -> Sum6/2
  Constant1/1 -> Matrix Concatenate/3
  Product7/1 -> i_q/1
  v_in/1 -> Selector1/1, Selector/1
  Gain4/1 -> Product/1
  i_d/1 -> Gain1/1, Sum/1  "id"
  Gain7/1 -> Product7/2
  Product1/1 -> Sum8/2
  Sum6/1 -> Gain5/1
  Gain1/1 -> Product1/2
  For Each Subsystem/1(Out1) -> i/1
  [omega_base] -> Selector8/1
  connected/1 -> Selector3/1
  i_q/1 -> Gain4/1, Sum1/1  "iq"
  Selector3/1 -> Product9/1, Product8/1
  Selector1/1 -> Product9/2
  Product6/1 -> i_d/1
  Selector/1 -> Product8/2
  Signal Specification/1 -> For Each Subsystem/1(In1)
  [omega_ref] -> Selector4/1  "omega"
  Selector4/1 -> Product1/1, Product/2
  Sum8/1 -> Gain7/1

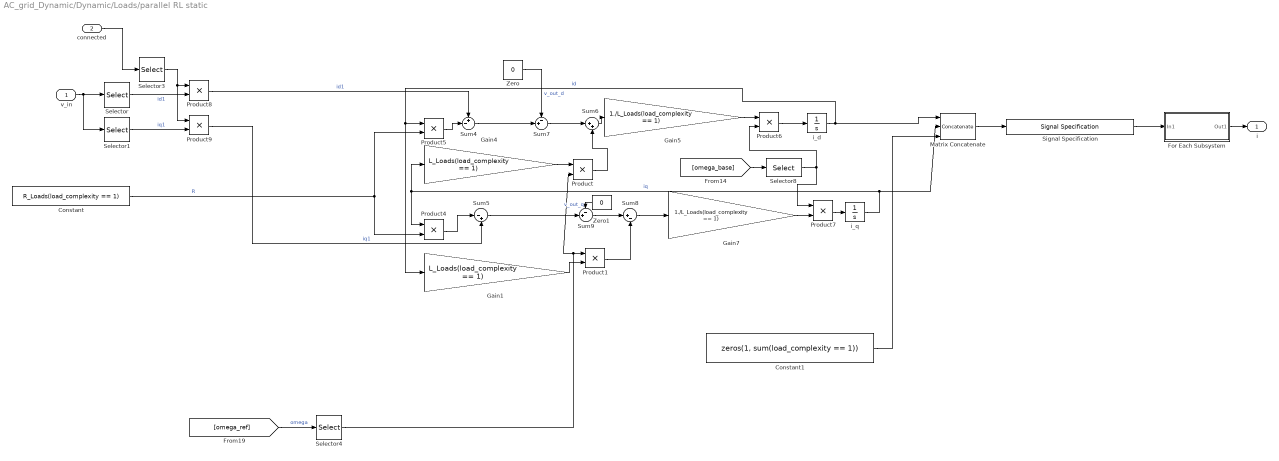
== system AC_grid_Dynamic/Dynamic/Loads/parallel RL static ==
  v_in : Inport
  connected : Inport  Port=2
  Constant : Constant  Value=R_Loads(load_complexity == 1)  VectorParams1D=off
  Constant1 : Constant  Value=zeros(1, sum(load_complexity == 1))  VectorParams1D=off
  For Each Subsystem : Subsystem  TreatAsAtomicUnit=on
  Gain1 : Gain  Gain=L_Loads(load_complexity == 1)
  Gain4 : Gain  Gain=L_Loads(load_complexity == 1)
  Gain5 : Gain  Gain=1./L_Loads(load_complexity == 1)
  Gain7 : Gain  Gain=1./L_Loads(load_complexity == 1)
  Matrix Concatenate : Concatenate  NumInputs=3  Mode=Multidimensional array
  Product{,1,4..9} (8 alike) : Product
  Selector : Selector  NumberOfDimensions=2  InputPortWidth=3  IndexOptions=Index vector (dialog),Index vector (dialog)  Indices=1,find(load_complexity == 1)  OutputSizes=1,1
  Selector1 : Selector  NumberOfDimensions=2  InputPortWidth=3  IndexOptions=Index vector (dialog),Index vector (dialog)  Indices=2,find(load_complexity == 1)  OutputSizes=1,1
  Selector3 : Selector  InputPortWidth=length(R_Loads)  IndexOptions=Index vector (dialog)  Indices=find(load_complexity == 1)  OutputSizes=1
  Selector4 : Selector  InputPortWidth=length(fref.ref_units)  IndexOptions=Index vector (dialog)  Indices=fref.loads(load_complexity == 1)  OutputSizes=1
  Selector8 : Selector  InputPortWidth=length(fref.ref_units)  IndexOptions=Index vector (dialog)  Indices=fref.loads(load_complexity == 1)  OutputSizes=1
  Signal Specification : SignalSpecification  Dimensions=[3 sum(load_complexity == 1)]
  Sum4 : Sum  Inputs=+-|
  Sum5 : Sum  Inputs=|-+
  Sum6 : Sum  Inputs=|++
  Sum7 : Sum  Inputs=-+|
  Sum8 : Sum  Inputs=|+-
  Sum9 : Sum  Inputs=-+|
  Zero : Constant  Value=0  OutDataTypeStr=Inherit: Inherit via back propagation
  Zero1 : Constant  Value=0  OutDataTypeStr=Inherit: Inherit via back propagation
  i_d : Integrator  InitialCondition=Grid_lf_op.op_report.Outputs(5).y(load_complexity == 1)
  i_q : Integrator  InitialCondition=Grid_lf_op.op_report.Outputs(6).y(load_complexity == 1)
  i : Outport
  wires:
  Selector1/1 -> Product9/2  "iq1"
  Selector3/1 -> Product8/1, Product9/1
  Selector/1 -> Product8/2  "id1"
  connected/1 -> Selector3/1
  Product6/1 -> i_d/1
  Gain5/1 -> Product6/1
  Gain7/1 -> Product7/2
  Product7/1 -> i_q/1
  Selector8/1 -> Product7/1, Product6/2
  [omega_base] -> Selector8/1
  Selector4/1 -> Product/2, Product1/1
  Constant/1 -> Product4/2, Product5/2  "R"
  Constant1/1 -> Matrix Concatenate/3
  Signal Specification/1 -> For Each Subsystem/1(In1)
  For Each Subsystem/1(Out1) -> i/1
  Product9/1 -> Sum5/2  "iq1"
  Product8/1 -> Sum4/1  "id1"
  Matrix Concatenate/1 -> Signal Specification/1
  Zero1/1 -> Sum9/1  "v_out_q"
  Zero/1 -> Sum7/1  "v_out_d"
  Sum9/1 -> Sum8/1
  Gain1/1 -> Product1/2
  i_q/1 -> Gain4/1, Product4/1, Matrix Concatenate/2  "iq"
  Sum5/1 -> Sum9/2
  Product4/1 -> Sum5/1
  Sum7/1 -> Sum6/1
  Gain4/1 -> Product/1
  Product1/1 -> Sum8/2
  Sum4/1 -> Sum7/2
  Sum8/1 -> Gain7/1
  Product/1 -> Sum6/2
  [omega_ref] -> Selector4/1  "omega"
  Sum6/1 -> Gain5/1
  i_d/1 -> Product5/1, Gain1/1, Matrix Concatenate/1  "id"
  Product5/1 -> Sum4/2
  v_in/1 -> Selector/1, Selector1/1

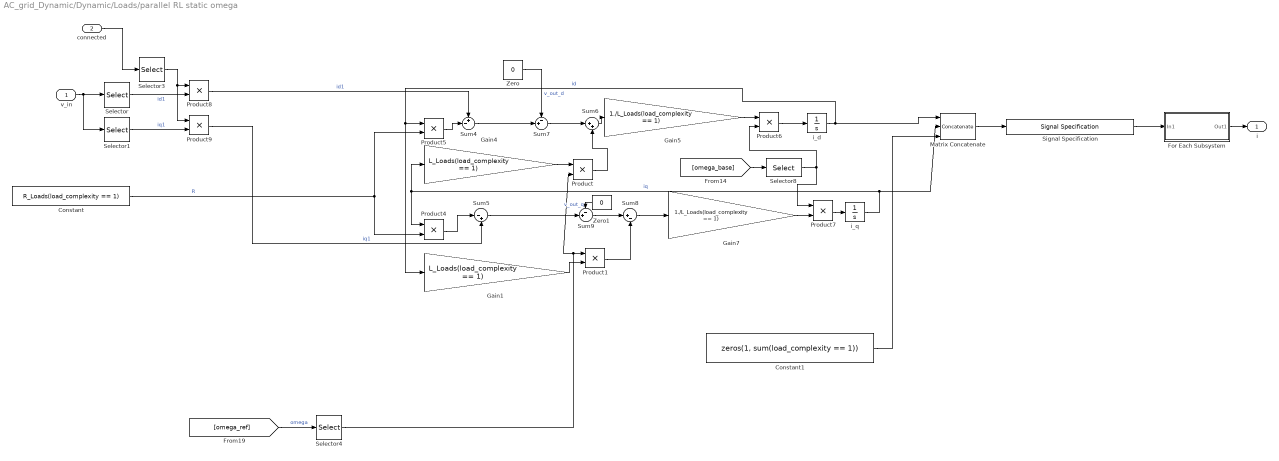
== system AC_grid_Dynamic/Dynamic/Loads/parallel RL static omega ==
  v_in : Inport
  connected : Inport  Port=2
  Constant : Constant  Value=R_Loads(load_complexity == 1)  VectorParams1D=off
  Constant1 : Constant  Value=zeros(1, sum(load_complexity == 1))  VectorParams1D=off
  For Each Subsystem : Subsystem  TreatAsAtomicUnit=on
  Gain1 : Gain  Gain=L_Loads(load_complexity == 1)
  Gain4 : Gain  Gain=L_Loads(load_complexity == 1)
  Gain5 : Gain  Gain=1./L_Loads(load_complexity == 1)
  Gain7 : Gain  Gain=1./L_Loads(load_complexity == 1)
  Matrix Concatenate : Concatenate  NumInputs=3  Mode=Multidimensional array
  Product{,1,4..9} (8 alike) : Product
  Selector : Selector  NumberOfDimensions=2  InputPortWidth=3  IndexOptions=Index vector (dialog),Index vector (dialog)  Indices=1,find(load_complexity == 1)  OutputSizes=1,1
  Selector1 : Selector  NumberOfDimensions=2  InputPortWidth=3  IndexOptions=Index vector (dialog),Index vector (dialog)  Indices=2,find(load_complexity == 1)  OutputSizes=1,1
  Selector3 : Selector  InputPortWidth=length(R_Loads)  IndexOptions=Index vector (dialog)  Indices=find(load_complexity == 1)  OutputSizes=1
  Selector4 : Selector  InputPortWidth=length(fref.ref_units)  IndexOptions=Index vector (dialog)  Indices=fref.loads(load_complexity == 1)  OutputSizes=1
  Selector8 : Selector  InputPortWidth=length(fref.ref_units)  IndexOptions=Index vector (dialog)  Indices=fref.loads(load_complexity == 1)  OutputSizes=1
  Signal Specification : SignalSpecification  Dimensions=[3 sum(load_complexity == 1)]
  Sum4 : Sum  Inputs=+-|
  Sum5 : Sum  Inputs=|-+
  Sum6 : Sum  Inputs=|++
  Sum7 : Sum  Inputs=-+|
  Sum8 : Sum  Inputs=|+-
  Sum9 : Sum  Inputs=-+|
  Zero : Constant  Value=0  OutDataTypeStr=Inherit: Inherit via back propagation
  Zero1 : Constant  Value=0  OutDataTypeStr=Inherit: Inherit via back propagation
  i_d : Integrator  InitialCondition=Grid_lf_op.op_report.Outputs(5).y(load_complexity == 1)
  i_q : Integrator  InitialCondition=Grid_lf_op.op_report.Outputs(6).y(load_complexity == 1)
  i : Outport
  wires:
  v_in/1 -> Selector1/1, Selector/1
  Product5/1 -> Sum4/2
  i_d/1 -> Matrix Concatenate/1, Gain1/1, Product5/1  "id"
  Sum6/1 -> Gain5/1
  [omega_ref] -> Selector4/1  "omega"
  Product/1 -> Sum6/2
  Sum8/1 -> Gain7/1
  Sum4/1 -> Sum7/2
  Product1/1 -> Sum8/2
  Gain4/1 -> Product/1
  Sum7/1 -> Sum6/1
  Product4/1 -> Sum5/1
  Sum5/1 -> Sum9/2
  i_q/1 -> Matrix Concatenate/2, Product4/1, Gain4/1  "iq"
  Gain1/1 -> Product1/2
  Sum9/1 -> Sum8/1
  Zero/1 -> Sum7/1  "v_out_d"
  Zero1/1 -> Sum9/1  "v_out_q"
  Matrix Concatenate/1 -> Signal Specification/1
  Product8/1 -> Sum4/1  "id1"
  Product9/1 -> Sum5/2  "iq1"
  For Each Subsystem/1(Out1) -> i/1
  Signal Specification/1 -> For Each Subsystem/1(In1)
  Constant1/1 -> Matrix Concatenate/3
  Constant/1 -> Product5/2, Product4/2  "R"
  Selector4/1 -> Product1/1, Product/2
  [omega_base] -> Selector8/1
  Selector8/1 -> Product6/2, Product7/1
  Product7/1 -> i_q/1
  Gain7/1 -> Product7/2
  Gain5/1 -> Product6/1
  Product6/1 -> i_d/1
  connected/1 -> Selector3/1
  Selector/1 -> Product8/2  "id1"
  Selector3/1 -> Product9/1, Product8/1
  Selector1/1 -> Product9/2  "iq1"

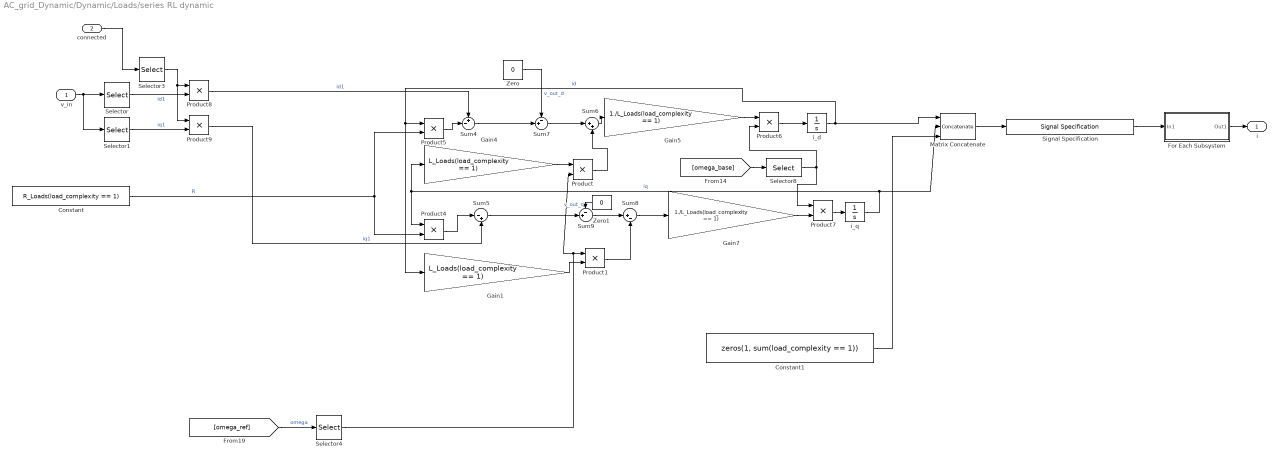
== system AC_grid_Dynamic/Dynamic/Loads/series RL dynamic ==
  v_in : Inport
  connected : Inport  Port=2
  Constant : Constant  Value=R_Loads(load_complexity == 1)  VectorParams1D=off
  Constant1 : Constant  Value=zeros(1, sum(load_complexity == 1))  VectorParams1D=off
  For Each Subsystem : Subsystem  TreatAsAtomicUnit=on
  Gain1 : Gain  Gain=L_Loads(load_complexity == 1)
  Gain4 : Gain  Gain=L_Loads(load_complexity == 1)
  Gain5 : Gain  Gain=1./L_Loads(load_complexity == 1)
  Gain7 : Gain  Gain=1./L_Loads(load_complexity == 1)
  Matrix Concatenate : Concatenate  NumInputs=3  Mode=Multidimensional array
  Product{,1,4..9} (8 alike) : Product
  Selector : Selector  NumberOfDimensions=2  InputPortWidth=3  IndexOptions=Index vector (dialog),Index vector (dialog)  Indices=1,find(load_complexity == 1)  OutputSizes=1,1
  Selector1 : Selector  NumberOfDimensions=2  InputPortWidth=3  IndexOptions=Index vector (dialog),Index vector (dialog)  Indices=2,find(load_complexity == 1)  OutputSizes=1,1
  Selector3 : Selector  InputPortWidth=length(R_Loads)  IndexOptions=Index vector (dialog)  Indices=find(load_complexity == 1)  OutputSizes=1
  Selector4 : Selector  InputPortWidth=length(fref.ref_units)  IndexOptions=Index vector (dialog)  Indices=fref.loads(load_complexity == 1)  OutputSizes=1
  Selector8 : Selector  InputPortWidth=length(fref.ref_units)  IndexOptions=Index vector (dialog)  Indices=fref.loads(load_complexity == 1)  OutputSizes=1
  Signal Specification : SignalSpecification  Dimensions=[3 sum(load_complexity == 1)]
  Sum4 : Sum  Inputs=+-|
  Sum5 : Sum  Inputs=|-+
  Sum6 : Sum  Inputs=|++
  Sum7 : Sum  Inputs=-+|
  Sum8 : Sum  Inputs=|+-
  Sum9 : Sum  Inputs=-+|
  Zero : Constant  Value=0  OutDataTypeStr=Inherit: Inherit via back propagation
  Zero1 : Constant  Value=0  OutDataTypeStr=Inherit: Inherit via back propagation
  i_d : Integrator  InitialCondition=Grid_lf_op.op_report.Outputs(5).y(load_complexity == 1)
  i_q : Integrator  InitialCondition=Grid_lf_op.op_report.Outputs(6).y(load_complexity == 1)
  i : Outport
  wires:
  Product7/1 -> i_q/1
  Product6/1 -> i_d/1
  Selector1/1 -> Product9/2  "iq1"
  Selector3/1 -> Product8/1, Product9/1
  Selector/1 -> Product8/2  "id1"
  connected/1 -> Selector3/1
  Gain5/1 -> Product6/1
  Gain7/1 -> Product7/2
  Selector8/1 -> Product7/1, Product6/2
  [omega_base] -> Selector8/1
  Selector4/1 -> Product/2, Product1/1
  Constant/1 -> Product4/2, Product5/2  "R"
  Constant1/1 -> Matrix Concatenate/3
  Signal Specification/1 -> For Each Subsystem/1(In1)
  For Each Subsystem/1(Out1) -> i/1
  Product9/1 -> Sum5/2  "iq1"
  Product8/1 -> Sum4/1  "id1"
  Matrix Concatenate/1 -> Signal Specification/1
  Zero1/1 -> Sum9/1  "v_out_q"
  Zero/1 -> Sum7/1  "v_out_d"
  Sum9/1 -> Sum8/1
  Gain1/1 -> Product1/2
  i_q/1 -> Gain4/1, Product4/1, Matrix Concatenate/2  "iq"
  Sum5/1 -> Sum9/2
  Product4/1 -> Sum5/1
  Sum7/1 -> Sum6/1
  Gain4/1 -> Product/1
  Product1/1 -> Sum8/2
  Sum4/1 -> Sum7/2
  Sum8/1 -> Gain7/1
  Product/1 -> Sum6/2
  [omega_ref] -> Selector4/1  "omega"
  Sum6/1 -> Gain5/1
  i_d/1 -> Product5/1, Gain1/1, Matrix Concatenate/1  "id"
  Product5/1 -> Sum4/2
  v_in/1 -> Selector/1, Selector1/1
